simulink model "studio2b"  (R2020a)
settings: Solver=ode45  StartTime=0.  StopTime=16  FixedStep=0.2  MaxStep=0.05  RelTol=1e-8  AbsTol=1e-8  EnableMultiTasking=on
settings Model: ExtModeTrigMode=oneshot  ExtModeArmWhenConnect=off  Creator=LEVIENKL  LastModifiedBy=New
settings SolverCC: AutoScaleAbsTol=off
settings DataIOCC: SaveFormat=Array  SignalLoggingSaveFormat=ModelDataLogs  SaveOutput=off  SaveTime=off  ReturnWorkspaceOutputs=off  SignalLoggingName=sigsOut
settings OptimizationCC: BlockReduction=off  BooleanDataType=off  ExpressionDepthLimit=2147483647  InitFltsAndDblsToZero=on  LifeSpan=inf
settings DebuggingCC: SaveWithParameterizedLinksMsg=none  UnderspecifiedInitializationDetection=Classic  MergeDetectMultiDrivingBlocksExec=none  SignalResolutionControl=TryResolveAllWithWarning  MultiTaskDSMMsg=warning  MultiTaskCondExecSysMsg=none  FcnCallInpInsideContextMsg=warning  AllowSymbolicDim=off  StateNameClashWarn=warning  SFUnexpectedBacktrackingDiag=warning  SFNoUnconditionalDefaultTransitionDiag=warning  SFExecutionAtInitializationDiag=none  ArithmeticOperatorsInVariantConditions=warning
settings HardwareCC: ProdBitPerPointer=32  ProdBitPerSizeT=32  ProdBitPerPtrDiffT=32  ProdLargestAtomicFloat=None  ProdIntDivRoundTo=Undefined  ProdEndianess=Unspecified  ProdWordSize=32  ProdHWDeviceType=32-bit Generic  TargetUnknown=on
settings ModelReferenceCC: PropagateSignalLabelsOutOfModel=off
settings SFSimCC: SimUseLocalCustomCode=off  CustomCodeUndefinedFunction=UseInterfaceOnly
settings RTWCC: RTWUseLocalCustomCode=off
settings CodeAppCC: StateflowObjectComments=on
settings GRTTargetCC: TargetFcnLib=ansi_tfl_tmw.mat  TargetLangStandard=C89/C90 (ANSI)  CombineOutputUpdateFcns=off  GRTInterface=on
settings ConfigComp: CovMetricSettings=dw  CovHtmlReporting=on  CovSaveCumulativeToWorkspaceVar=on  CovSaveSingleToWorkspaceVar=on  CovExternalEMLEnable=off  CovSFcnEnable=off

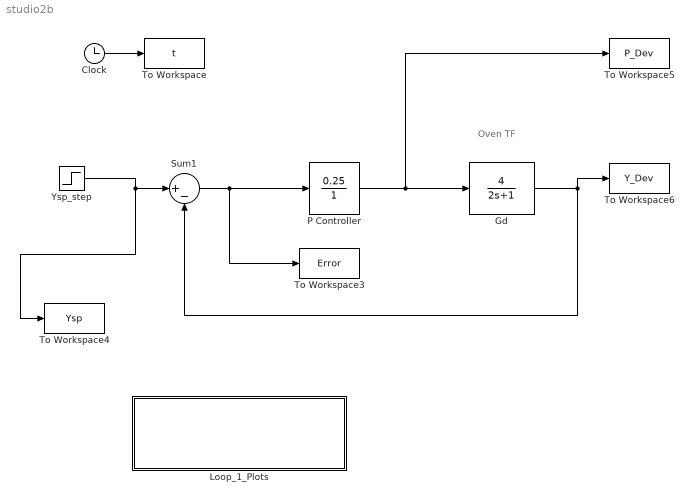
== system studio2b ==
  note: Oven TF
  Clock : Clock
  Gd : TransferFcn  Numerator=[4]  Denominator=[2 1]
  Loop_1_Plots : Subsystem  mask(Y,U,E Plots - Loop 1){}
      settings: OpenFcn=YPEplots
      mask Help: This block loop #1 Y,U,Error in 3x1 Figure Window.
      mask Display: disp('After Loop 1 Simulation:\n Double Click for Y, P, Error Plots\n (uses YPEplots.p)')
  P Controller : TransferFcn  Numerator=[0.25]  Denominator=[1]
  Sum1 : Sum  Inputs=|+-  InputSameDT=on  SaturateOnIntegerOverflow=on  OutDataTypeStr=Inherit: Same as first input
  To Workspace : ToWorkspace  VariableName=t  SampleTime=-1
  To Workspace3 : ToWorkspace  VariableName=Error  SampleTime=-1
  To Workspace4 : ToWorkspace  VariableName=Ysp  SampleTime=-1
  To Workspace5 : ToWorkspace  VariableName=P_Dev  SampleTime=-1
  To Workspace6 : ToWorkspace  VariableName=Y_Dev  SampleTime=-1
  Ysp_step : Step  Time=2  After=10  SampleTime=0
      settings: AttributesFormatString=%<Before> to %<After>\nat %<Time>
  wires:
  Clock/1 -> To Workspace/1
  Gd/1 -> To Workspace6/1, Sum1/2
  Ysp_step/1 -> To Workspace4/1, Sum1/1
  Sum1/1 -> To Workspace3/1, P Controller/1
  P Controller/1 -> To Workspace5/1, Gd/1

== system studio2b/Loop_1_Plots ==
